simulink model "q3"  (R2018b)
settings: Solver=FixedStepAuto  StartTime=0.0  StopTime=10.0  FixedStep=0.00001  RelTol=1e-3
settings Model: Creator=hp  LastModifiedBy=hp
settings DebuggingCC: LibraryContextMissingDiagnostic=none
settings SFSimCC: SimUseLocalCustomCode=off
settings RTWCC: RTWUseLocalCustomCode=off

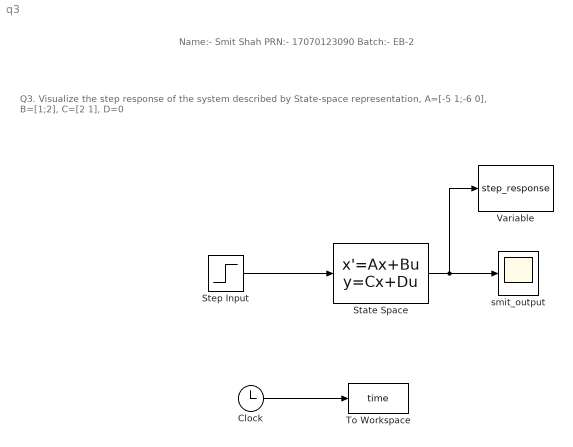
== system q3 ==
  note: Name:- Smit Shah PRN:- 17070123090 Batch:- EB-2
  note: Q3. Visualize the step response of the system described by State-space representation, A=[-5 1;-6 0], B=[1;2], C=[2 1], D=0
  Clock : Clock
  State Space : StateSpace  A=[-5 1;-6 0]  B=[1;2]  C=[2 1]  D=0  InitialCondition=0
  Step Input : Step  Time=0  SampleTime=0
  To Workspace : ToWorkspace  VariableName=time  SampleTime=-1
  Variable : ToWorkspace  VariableName=step_response  SampleTime=-1
  smit_output : Scope
  wires:
  State Space/1 -> Variable/1, smit_output/1
  Step Input/1 -> State Space/1
  Clock/1 -> To Workspace/1
